simulink model "neoArm_control"  (R2023a)
settings: Solver=VariableStepAuto  StartTime=0.0  StopTime=48  FixedStep=0.01  RelTol=1e-3
values from neighbouring files (symbols this model uses):
  dq0 = [0;0;0;0;0]    [neoArm_main.m]
  K = [1000  900]    [neoArm_main.m]
  objectPos = 0.2    [neoArm_main.m]
  orientations = pi/2*[ones(length(temp1),1) zeros(length(temp1),1) zeros(length(temp1),1)]'    [nesneTakip.m]
  q0 = [0;0;0;0;0]    [neoArm_main.m]
  refPos = 0.0    (= 0)    [neoArm_main.m]
  ts = 0.02    [neoArm_main.m]
  waypoints = temp1'    [nesneTakip.m]
  waypointTimes = linspace(0,tDuration,sayi)    [neoArm_main.m]
  weights = [0 0 0 1 1 1]    [neoArm_main.m]
undefined symbols (not defined in the file or in its folder): eul2tform, trvec2tform, X, Y, Z
libraries: sm_lib x147, nesl_utility x52, robotmaniplib x7, robotcorelib x5, simulink x2
(part 1 of 4)
settings Model: PacingRate=0.110000  Creator=guven  LastModifiedBy=guven
settings SolverCC: ZeroCrossAlgorithm=Adaptive
settings DataIOCC: ReturnWorkspaceOutputs=off
settings DebuggingCC: IgnoredZcDiagnostic=none
settings ModelReferenceCC: EnableRefExpFcnMdlSchedulingChecks=on

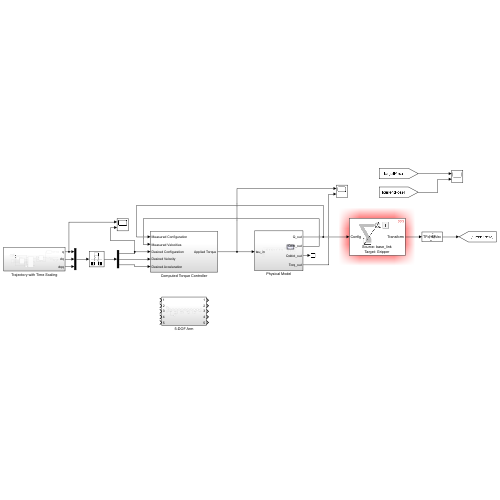
[thumbnail: Simulink's stored preview of the top-level diagram]
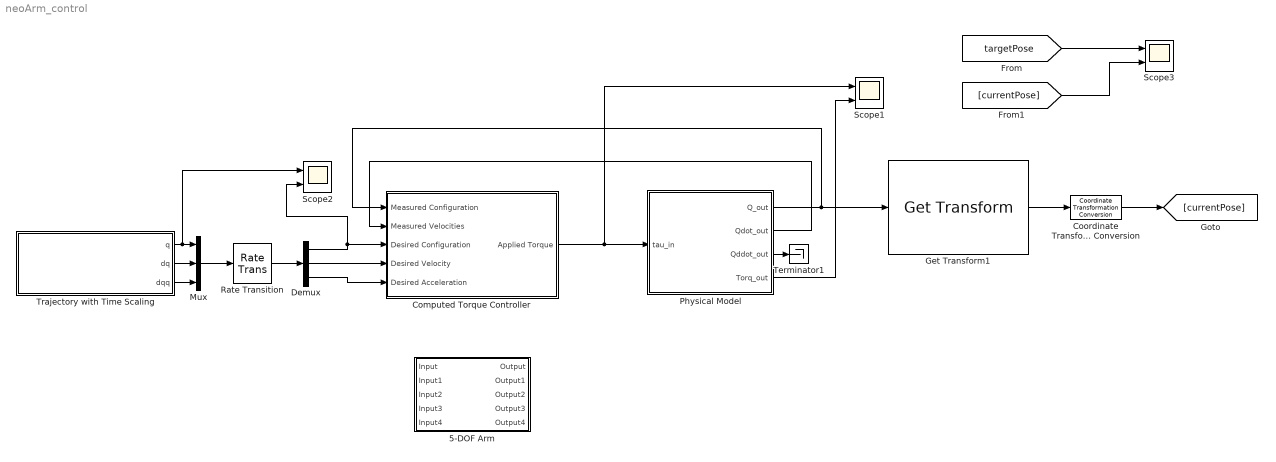
== system neoArm_control ==
  5-DOF Arm : Subsystem
  Computed Torque Controller : Subsystem
  Coordinate Transformation Conversion : robotcorelib/Coordinate Transformation Conversion  InputRepresentation=Homogeneous Transformation  InputEulerSequence=ZYX  ShowTrVecInputPort=on  OutputRepresentation=Translation Vector  OutputEulerSequence=ZYX  ShowTrVecOutputPort=on  SimulateUsing=Interpreted execution
      settings: LibrarySourceBlock=navlib/Utilities/Coordinate Transformation Conversion
  Demux : Demux  Outputs=3
  Get Transform1 : robotmaniplib/Get Transform  RigidBodyTree=gen3  SourceBody=base_link  TargetBody=Gripper  SimulateUsing=Interpreted execution
  Mux : Mux  Inputs=3
  Physical Model : Subsystem
  Rate Transition : RateTransition
  Scope1 : Scope  NumInputPorts=2
  Scope2 : Scope  NumInputPorts=2
  Scope3 : Scope  NumInputPorts=2
  Terminator1 : Terminator
  Trajectory with Time Scaling : Subsystem
  wires:
  Physical Model/2(Qdot_out) -> Computed Torque Controller/2(Measured Velocities)
  Get Transform1/1 -> Coordinate Transformation Conversion/1
  Physical Model/4(Torq_out) -> Scope1/2
  [targetPose] -> Scope3/1
  [currentPose] -> Scope3/2
  Coordinate Transformation Conversion/1 -> [currentPose]
  Physical Model/1(Q_out) -> Computed Torque Controller/1(Measured Configuration), Get Transform1/1
  Physical Model/3(Qddot_out) -> Terminator1/1
  Computed Torque Controller/1(Applied Torque) -> Physical Model/1(tau_in), Scope1/1
  Trajectory with Time Scaling/1(q) -> Scope2/1, Mux/1
  Trajectory with Time Scaling/3(dqq) -> Mux/3
  Trajectory with Time Scaling/2(dq) -> Mux/2
  Mux/1 -> Rate Transition/1
  Rate Transition/1 -> Demux/1
  Demux/1 -> Scope2/2, Computed Torque Controller/3(Desired Configuration)
  Demux/2 -> Computed Torque Controller/4(Desired Velocity)
  Demux/3 -> Computed Torque Controller/5(Desired Acceleration)

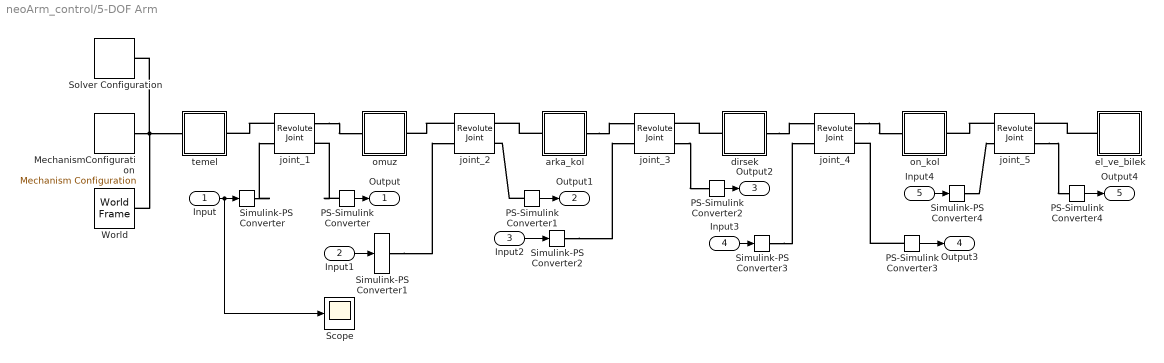
== system neoArm_control/5-DOF Arm ==
  Input : Inport
  Input1 : Inport  Port=2
  Input2 : Inport  Port=3
  Input3 : Inport  Port=4
  Input4 : Inport  Port=5
  MechanismConfiguration : sm_lib/Utilities/Mechanism Configuration  UniformGravity=Constant  GravityVector=[0 0 -9.80665]  GravityVectorUnits=m/s^2  LinearizationDelta=0.001  JointModeTransitionNonlinearIterations=2
  PS-Simulink Converter{,1..4} (5 alike) : nesl_utility/PS-Simulink Converter  PhysicalDomain=network_engine_domain  SubClassName=ps_output  LeftPortType=input  RightPortType=output  PseudoPeriodic=off  Frequencies=[]  VectorFormat=inherit  Unit=inherit  AffineConversion=off
  Scope : Scope
  Simulink-PS Converter{,2..4} (4 alike) : nesl_utility/Simulink-PS Converter  PhysicalDomain=network_engine_domain  SubClassName=ps_input  LeftPortType=input  RightPortType=output  PseudoPeriodic=off  Frequencies=[]  NoiseDistribution=none  NoiseParameters=[]  Unit=rad  AffineConversion=off  FilteringAndDerivatives=filter  SimscapeFilterOrder=2  InputFilterTimeConstant=0.001  UdotUserProvided=0
  Simulink-PS Converter1 : nesl_utility/Simulink-PS Converter  PhysicalDomain=network_engine_domain  SubClassName=ps_input  LeftPortType=input  RightPortType=output  PseudoPeriodic=off  Frequencies=[]  NoiseDistribution=none  NoiseParameters=[]  Unit=rad  AffineConversion=off  FilteringAndDerivatives=filter  SimscapeFilterOrder=2  InputFilterTimeConstant=0.001  UdotUserProvided=2
  Solver Configuration : nesl_utility/Solver Configuration  PhysicalDomain=network_engine_domain  SubClassName=solver  LeftPortType=input  RightPortType=generic  Tones=[]  Harmonics=[]  SimulateNoise=off  Profile=off  UseLocalSampling=off  EnableSwitchedLinearOptims=on  FrequencyDomain=off  UseCCode=off  RelTol=0.001  AbsTol=0.001  MinStep=1e-09  ToWorkspace=off  RevertToSquareIcSolve=off  NumHomotopyIterations=100  PhasorMode=off  PhasorModeNumHarmonics=1  ConsistencySolver=NEWTON_XTOL_AFTER_FTOL  IndexReductionMethod=DerivativeReplacement  DoDC=off  ResidualTolerance=1e-09  ConsistencyTolSource=GLOBAL  ConsistencyAbsTol=0.001  ConsistencyRelTol=0.001  ConsistencyTolFactor=0.001  UseLocalSolver=off  LocalSolverChoice=NE_BACKWARD_EULER_ADVANCER  ResolveIndetEquations=on  FunctionEvalNumThread=1  LocalSolverSampleTime=0.001  DoFixedCost=off  MaxNonlinIter=3  MaxModeIter=2  ComputeImpulses=off  ImpulseIterations=2  LinearAlgebra=auto  LinearAlgebraNumThread=0  EquationFormulation=NE_TIME_EF  DelaysMemoryBudget=1024  AutomaticFiltering=on  FilteringTimeConstant=0.001  PartitionStorageMethod=AS_NEEDED  PartitionMemoryBudget=1024  PartitionMethod=ROBUST
  World : sm_lib/Frames and Transforms/World Frame
  arka_kol : Subsystem
  dirsek : Subsystem
  el_ve_bilek : Subsystem
  joint_{1..5} (5 alike) : sm_lib/Joints/Revolute Joint  JointMode=Normal  SenseConstraintForce=off  SenseConstraintForceX=off  SenseConstraintForceY=off  SenseConstraintForceZ=off  SenseConstraintTorque=off  SenseConstraintTorqueX=off  SenseConstraintTorqueY=off  SenseConstraintTorqueZ=off  SenseTotalForce=off  SenseTotalForceX=off  SenseTotalForceY=off  SenseTotalForceZ=off  SenseTotalTorque=off  SenseTotalTorqueX=off  SenseTotalTorqueY=off  SenseTotalTorqueZ=off  CompositeWrenchDir=FollowerOnBase  CompositeWrenchFrame=BaseFrame  EquilibriumPosition=0  EquilibriumPositionUnits=deg  SpringStiffness=0  SpringStiffnessUnits=N*m/deg  DampingCoefficient=0  DampingCoefficientUnits=kg*m^2/(rad*s)  TorqueActuationMode=ComputedTorque  MotionActuationMode=InputMotion  SensePosition=on  SenseVelocity=off  SenseAcceleration=off  SenseTorqueForce=off  SenseLowerLimitTorqueForce=off  SenseUpperLimitTorqueForce=off  LowerLimitSpecify=off  LowerLimitBound=0  LowerLimitBoundUnits=rad  LowerLimitStiffness=1e4  LowerLimitStiffnessUnits=N*m/deg  LowerLimitDamping=10  LowerLimitDampingUnits=N*m/(deg/s)  LowerLimitTransitionRegionWidth=0.1  LowerLimitTransitionRegionWidthUnits=deg  UpperLimitSpecify=off  UpperLimitBound=0  UpperLimitBoundUnits=rad  UpperLimitStiffness=1e4  UpperLimitStiffnessUnits=N*m/deg  UpperLimitDamping=10  UpperLimitDampingUnits=N*m/(deg/s)  UpperLimitTransitionRegionWidth=0.1  UpperLimitTransitionRegionWidthUnits=deg  PositionTargetSpecify=off  PositionTargetPriority=High  PositionTargetValue=0  PositionTargetValueUnits=deg  VelocityTargetSpecify=off  VelocityTargetPriority=High  VelocityTargetValue=0  VelocityTargetValueUnits=deg/s
  omuz : Subsystem
  on_kol : Subsystem
  temel : Subsystem
  Output : Outport
  Output1 : Outport  Port=2
  Output2 : Outport  Port=3
  Output3 : Outport  Port=4
  Output4 : Outport  Port=5
  wires:
  Input1/1 -> Simulink-PS Converter1/1
  Input2/1 -> Simulink-PS Converter2/1
  Input3/1 -> Simulink-PS Converter3/1
  Input4/1 -> Simulink-PS Converter4/1
  PS-Simulink Converter/1 -> Output/1
  PS-Simulink Converter1/1 -> Output1/1
  PS-Simulink Converter2/1 -> Output2/1
  PS-Simulink Converter3/1 -> Output3/1
  PS-Simulink Converter4/1 -> Output4/1
  Input/1 -> Scope/1, Simulink-PS Converter/1
  connections:
  joint_5/LConn1 -- on_kol/RConn1
  arka_kol/LConn1 -- joint_2/RConn1
  joint_2/LConn1 -- omuz/RConn1
  dirsek/RConn1 -- joint_4/LConn1
  MechanismConfiguration/RConn1 -- Solver Configuration/RConn1 -- temel/LConn1 -- World/RConn1
  arka_kol/RConn1 -- joint_3/LConn1
  joint_4/RConn1 -- on_kol/LConn1
  dirsek/LConn1 -- joint_3/RConn1
  joint_1/RConn1 -- omuz/LConn1
  joint_1/LConn1 -- temel/RConn1
  el_ve_bilek/LConn1 -- joint_5/RConn1
  Simulink-PS Converter1/RConn1 -- joint_2/LConn2
  PS-Simulink Converter/LConn1 -- joint_1/RConn2
  PS-Simulink Converter1/LConn1 -- joint_2/RConn2
  joint_3/RConn2 -- PS-Simulink Converter2/LConn1
  PS-Simulink Converter3/LConn1 -- joint_4/RConn2
  joint_5/RConn2 -- PS-Simulink Converter4/LConn1
  Simulink-PS Converter/RConn1 -- joint_1/LConn2
  Simulink-PS Converter2/RConn1 -- joint_3/LConn2
  Simulink-PS Converter3/RConn1 -- joint_4/LConn2
  Simulink-PS Converter4/RConn1 -- joint_5/LConn2

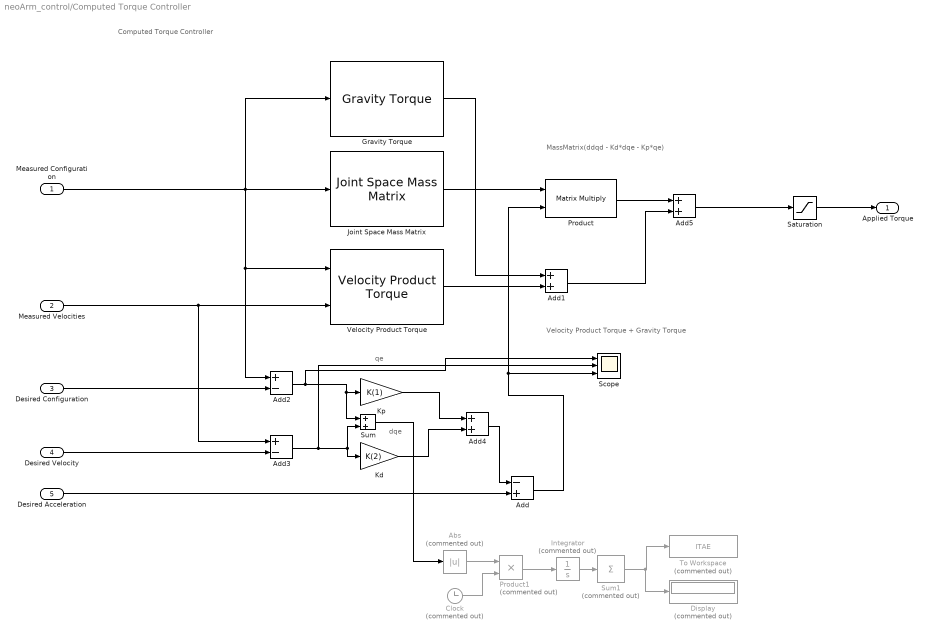
== system neoArm_control/Computed Torque Controller ==
  note: Computed Torque Controller
  note: MassMatrix(ddqd - Kd*dqe - Kp*qe)
  note: Velocity Product Torque + Gravity Torque
  note: dqe
  note: qe
  Measured Configuration : Inport
  Measured Velocities : Inport  Port=2
  Desired Configuration : Inport  Port=3
  Desired Velocity : Inport  Port=4
  Desired Acceleration : Inport  Port=5
  Abs : Abs  Commented=on  SaturateOnIntegerOverflow=off
  Add : Sum  Inputs=-+
  Add1 : Sum
  Add2 : Sum  Inputs=+-
  Add3 : Sum  Inputs=+-
  Add4 : Sum
  Add5 : Sum
  Clock : Clock  Commented=on
  Display : Display  Commented=on
  Gravity Torque : robotmaniplib/Gravity Torque  RigidBodyTree=gen3  SimulateUsing=Interpreted execution
  Integrator : Integrator  Commented=on
  Joint Space Mass Matrix : robotmaniplib/Joint Space Mass Matrix  RigidBodyTree=gen3  SimulateUsing=Interpreted execution
  Kd : Gain  Gain=K(2)
  Kp : Gain  Gain=K(1)
  Product : Product  Multiplication=Matrix(*)
  Product1 : Product  Commented=on
  Saturation : Saturate  UpperLimit=100  LowerLimit=-100
  Scope : Scope  NumInputPorts=3
  Sum : Sum
  Sum1 : Sum  Commented=on  Inputs=+
  To Workspace : ToWorkspace  Commented=on  VariableName=ITAE  SampleTime=-1
      settings: Save2DSignal=2-D array (concatenate along first dimension)
  Velocity Product Torque : robotmaniplib/Velocity Product Torque  RigidBodyTree=gen3  SimulateUsing=Interpreted execution
  Applied Torque : Outport  VectorParamsAs1DForOutWhenUnconnected=off
  wires:
  Add5/1 -> Saturation/1
  Velocity Product Torque/1 -> Add1/2
  Gravity Torque/1 -> Add1/1
  Add1/1 -> Add5/2
  Product/1 -> Add5/1
  Kd/1 -> Add4/2
  Kp/1 -> Add4/1
  Add3/1 -> Scope/2, Kd/1, Sum/2
  Add2/1 -> Scope/1, Sum/1, Kp/1
  Desired Configuration/1 -> Add2/2
  Add/1 -> Product/2, Scope/3
  Desired Acceleration/1 -> Add/2
  Add4/1 -> Add/1
  Measured Velocities/1 -> Velocity Product Torque/2, Add3/1
  Measured Configuration/1 -> Add2/1, Velocity Product Torque/1, Gravity Torque/1, Joint Space Mass Matrix/1
  Joint Space Mass Matrix/1 -> Product/1
  Desired Velocity/1 -> Add3/2
  Sum/1 -> Abs/1
  Clock/1 -> Product1/2
  Abs/1 -> Product1/1
  Product1/1 -> Integrator/1
  Integrator/1 -> Sum1/1
  Sum1/1 -> Display/1, To Workspace/1
  Saturation/1 -> Applied Torque/1

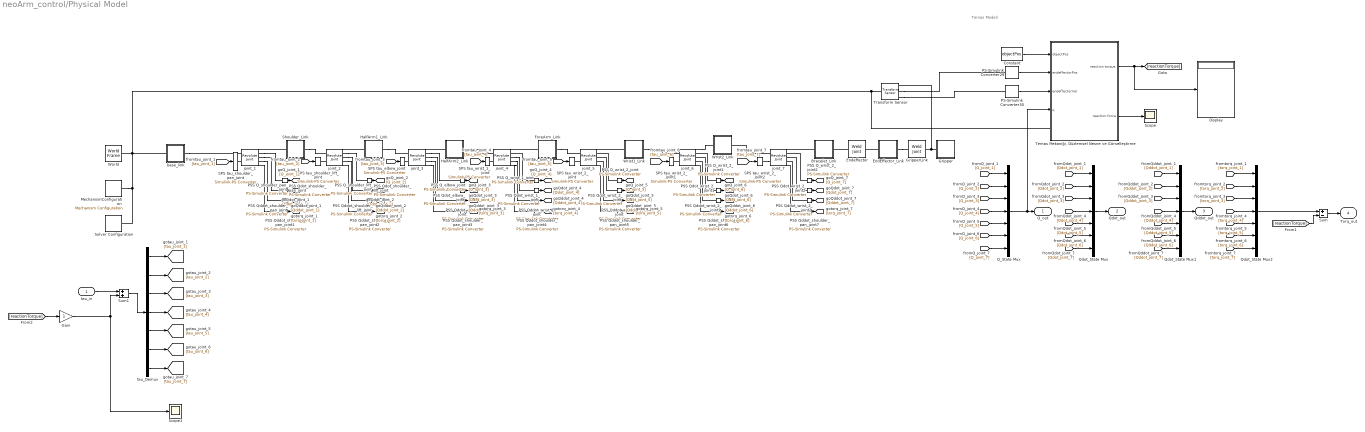
== system neoArm_control/Physical Model ==
  note: Temas Modeli
  tau_in : Inport
  Bracelet_Link : Subsystem
  Constant : Constant  Value=objectPos
  Display : Display
  EndEffector_Link : Subsystem
  Endeffector : sm_lib/Joints/Weld Joint  JointMode=Normal  SenseConstraintForce=off  SenseConstraintForceX=off  SenseConstraintForceY=off  SenseConstraintForceZ=off  SenseConstraintTorque=off  SenseConstraintTorqueX=off  SenseConstraintTorqueY=off  SenseConstraintTorqueZ=off  SenseTotalForce=off  SenseTotalForceX=off  SenseTotalForceY=off  SenseTotalForceZ=off  SenseTotalTorque=off  SenseTotalTorqueX=off  SenseTotalTorqueY=off  SenseTotalTorqueZ=off  CompositeWrenchDir=FollowerOnBase  CompositeWrenchFrame=BaseFrame
  ForeArm_Link : Subsystem
  Gain : Gain
  Gripper : Subsystem
  GripperLink : sm_lib/Joints/Weld Joint  JointMode=Normal  SenseConstraintForce=off  SenseConstraintForceX=off  SenseConstraintForceY=off  SenseConstraintForceZ=off  SenseConstraintTorque=off  SenseConstraintTorqueX=off  SenseConstraintTorqueY=off  SenseConstraintTorqueZ=off  SenseTotalForce=off  SenseTotalForceX=off  SenseTotalForceY=off  SenseTotalForceZ=off  SenseTotalTorque=off  SenseTotalTorqueX=off  SenseTotalTorqueY=off  SenseTotalTorqueZ=off  CompositeWrenchDir=FollowerOnBase  CompositeWrenchFrame=BaseFrame
  HalfArm1_Link : Subsystem
  HalfArm2_Link : Subsystem
  MechanismConfiguration : sm_lib/Utilities/Mechanism Configuration  UniformGravity=Constant  GravityVector=[0, 0, 0]  GravityVectorUnits=m/s^2  LinearizationDelta=0.001  JointModeTransitionNonlinearIterations=2
  PS-Simulink Converter29 : nesl_utility/PS-Simulink Converter  PhysicalDomain=network_engine_domain  SubClassName=ps_output  LeftPortType=input  RightPortType=output  PseudoPeriodic=off  Frequencies=[]  VectorFormat=1-D array  Unit=1  AffineConversion=off
  PS-Simulink Converter30 : nesl_utility/PS-Simulink Converter  PhysicalDomain=network_engine_domain  SubClassName=ps_output  LeftPortType=input  RightPortType=output  PseudoPeriodic=off  Frequencies=[]  VectorFormat=1-D array  Unit=1  AffineConversion=off
  PSS Q_elbow_joint : nesl_utility/PS-Simulink Converter  PhysicalDomain=network_engine_domain  SubClassName=ps_output  LeftPortType=input  RightPortType=output  PseudoPeriodic=off  Frequencies=[]  VectorFormat=inherit  Unit=inherit  AffineConversion=off
  PSS Q_shoulder_lift_joint : nesl_utility/PS-Simulink Converter  PhysicalDomain=network_engine_domain  SubClassName=ps_output  LeftPortType=input  RightPortType=output  PseudoPeriodic=off  Frequencies=[]  VectorFormat=inherit  Unit=inherit  AffineConversion=off
  PSS Q_shoulder_pan_joint : nesl_utility/PS-Simulink Converter  PhysicalDomain=network_engine_domain  SubClassName=ps_output  LeftPortType=input  RightPortType=output  PseudoPeriodic=off  Frequencies=[]  VectorFormat=inherit  Unit=inherit  AffineConversion=off
  PSS Q_wrist_1_joint : nesl_utility/PS-Simulink Converter  PhysicalDomain=network_engine_domain  SubClassName=ps_output  LeftPortType=input  RightPortType=output  PseudoPeriodic=off  Frequencies=[]  VectorFormat=inherit  Unit=inherit  AffineConversion=off
  PSS Q_wrist_2_joint : nesl_utility/PS-Simulink Converter  PhysicalDomain=network_engine_domain  SubClassName=ps_output  LeftPortType=input  RightPortType=output  PseudoPeriodic=off  Frequencies=[]  VectorFormat=inherit  Unit=inherit  AffineConversion=off
  PSS Q_wrist_2_joint1 : nesl_utility/PS-Simulink Converter  PhysicalDomain=network_engine_domain  SubClassName=ps_output  LeftPortType=input  RightPortType=output  PseudoPeriodic=off  Frequencies=[]  VectorFormat=inherit  Unit=inherit  AffineConversion=off
  PSS Q_wrist_2_joint2 : nesl_utility/PS-Simulink Converter  PhysicalDomain=network_engine_domain  SubClassName=ps_output  LeftPortType=input  RightPortType=output  PseudoPeriodic=off  Frequencies=[]  VectorFormat=inherit  Unit=inherit  AffineConversion=off
  PSS Qddot_elbow_joint : nesl_utility/PS-Simulink Converter  PhysicalDomain=network_engine_domain  SubClassName=ps_output  LeftPortType=input  RightPortType=output  PseudoPeriodic=off  Frequencies=[]  VectorFormat=inherit  Unit=inherit  AffineConversion=off
  PSS Qddot_shoulder_lift_joint : nesl_utility/PS-Simulink Converter  PhysicalDomain=network_engine_domain  SubClassName=ps_output  LeftPortType=input  RightPortType=output  PseudoPeriodic=off  Frequencies=[]  VectorFormat=inherit  Unit=inherit  AffineConversion=off
  PSS Qddot_shoulder_pan_joint{,1..7} (8 alike) : nesl_utility/PS-Simulink Converter  PhysicalDomain=network_engine_domain  SubClassName=ps_output  LeftPortType=input  RightPortType=output  PseudoPeriodic=off  Frequencies=[]  VectorFormat=inherit  Unit=inherit  AffineConversion=off
  PSS Qddot_wrist_1_joint : nesl_utility/PS-Simulink Converter  PhysicalDomain=network_engine_domain  SubClassName=ps_output  LeftPortType=input  RightPortType=output  PseudoPeriodic=off  Frequencies=[]  VectorFormat=inherit  Unit=inherit  AffineConversion=off
  PSS Qddot_wrist_2_joint : nesl_utility/PS-Simulink Converter  PhysicalDomain=network_engine_domain  SubClassName=ps_output  LeftPortType=input  RightPortType=output  PseudoPeriodic=off  Frequencies=[]  VectorFormat=inherit  Unit=inherit  AffineConversion=off
  PSS Qddot_wrist_2_joint1 : nesl_utility/PS-Simulink Converter  PhysicalDomain=network_engine_domain  SubClassName=ps_output  LeftPortType=input  RightPortType=output  PseudoPeriodic=off  Frequencies=[]  VectorFormat=inherit  Unit=inherit  AffineConversion=off
  PSS Qddot_wrist_2_joint2 : nesl_utility/PS-Simulink Converter  PhysicalDomain=network_engine_domain  SubClassName=ps_output  LeftPortType=input  RightPortType=output  PseudoPeriodic=off  Frequencies=[]  VectorFormat=inherit  Unit=inherit  AffineConversion=off
  PSS Qdot_elbow_joint : nesl_utility/PS-Simulink Converter  PhysicalDomain=network_engine_domain  SubClassName=ps_output  LeftPortType=input  RightPortType=output  PseudoPeriodic=off  Frequencies=[]  VectorFormat=inherit  Unit=inherit  AffineConversion=off
  PSS Qdot_shoulder_lift_joint : nesl_utility/PS-Simulink Converter  PhysicalDomain=network_engine_domain  SubClassName=ps_output  LeftPortType=input  RightPortType=output  PseudoPeriodic=off  Frequencies=[]  VectorFormat=inherit  Unit=inherit  AffineConversion=off
  PSS Qdot_shoulder_pan_joint : nesl_utility/PS-Simulink Converter  PhysicalDomain=network_engine_domain  SubClassName=ps_output  LeftPortType=input  RightPortType=output  PseudoPeriodic=off  Frequencies=[]  VectorFormat=inherit  Unit=inherit  AffineConversion=off
  PSS Qdot_wrist_1_joint : nesl_utility/PS-Simulink Converter  PhysicalDomain=network_engine_domain  SubClassName=ps_output  LeftPortType=input  RightPortType=output  PseudoPeriodic=off  Frequencies=[]  VectorFormat=inherit  Unit=inherit  AffineConversion=off
  PSS Qdot_wrist_2_joint : nesl_utility/PS-Simulink Converter  PhysicalDomain=network_engine_domain  SubClassName=ps_output  LeftPortType=input  RightPortType=output  PseudoPeriodic=off  Frequencies=[]  VectorFormat=inherit  Unit=inherit  AffineConversion=off
  PSS Qdot_wrist_2_joint1 : nesl_utility/PS-Simulink Converter  PhysicalDomain=network_engine_domain  SubClassName=ps_output  LeftPortType=input  RightPortType=output  PseudoPeriodic=off  Frequencies=[]  VectorFormat=inherit  Unit=inherit  AffineConversion=off
  PSS Qdot_wrist_2_joint2 : nesl_utility/PS-Simulink Converter  PhysicalDomain=network_engine_domain  SubClassName=ps_output  LeftPortType=input  RightPortType=output  PseudoPeriodic=off  Frequencies=[]  VectorFormat=inherit  Unit=inherit  AffineConversion=off
  Q_State Mux : Mux  Inputs=7
  Qdot_State Mux : Mux  Inputs=7
  Qdot_State Mux1 : Mux  Inputs=7
  Qdot_State Mux2 : Mux  Inputs=7
  SPS tau_elbow_joint : nesl_utility/Simulink-PS Converter  PhysicalDomain=network_engine_domain  SubClassName=ps_input  LeftPortType=input  RightPortType=output  PseudoPeriodic=off  Frequencies=[]  NoiseDistribution=none  NoiseParameters=[]  Unit=1  AffineConversion=off  FilteringAndDerivatives=filter  SimscapeFilterOrder=2  InputFilterTimeConstant=0.001  UdotUserProvided=0
  SPS tau_shoulder_lift_joint : nesl_utility/Simulink-PS Converter  PhysicalDomain=network_engine_domain  SubClassName=ps_input  LeftPortType=input  RightPortType=output  PseudoPeriodic=off  Frequencies=[]  NoiseDistribution=none  NoiseParameters=[]  Unit=1  AffineConversion=off  FilteringAndDerivatives=filter  SimscapeFilterOrder=2  InputFilterTimeConstant=0.001  UdotUserProvided=0
  SPS tau_shoulder_pan_joint : nesl_utility/Simulink-PS Converter  PhysicalDomain=network_engine_domain  SubClassName=ps_input  LeftPortType=input  RightPortType=output  PseudoPeriodic=off  Frequencies=[]  NoiseDistribution=none  NoiseParameters=[]  Unit=1  AffineConversion=off  FilteringAndDerivatives=filter  SimscapeFilterOrder=2  InputFilterTimeConstant=0.001  UdotUserProvided=0
  SPS tau_wrist_1_joint : nesl_utility/Simulink-PS Converter  PhysicalDomain=network_engine_domain  SubClassName=ps_input  LeftPortType=input  RightPortType=output  PseudoPeriodic=off  Frequencies=[]  NoiseDistribution=none  NoiseParameters=[]  Unit=1  AffineConversion=off  FilteringAndDerivatives=filter  SimscapeFilterOrder=2  InputFilterTimeConstant=0.001  UdotUserProvided=0
  SPS tau_wrist_2_joint : nesl_utility/Simulink-PS Converter  PhysicalDomain=network_engine_domain  SubClassName=ps_input  LeftPortType=input  RightPortType=output  PseudoPeriodic=off  Frequencies=[]  NoiseDistribution=none  NoiseParameters=[]  Unit=1  AffineConversion=off  FilteringAndDerivatives=filter  SimscapeFilterOrder=2  InputFilterTimeConstant=0.001  UdotUserProvided=0
  SPS tau_wrist_2_joint1 : nesl_utility/Simulink-PS Converter  PhysicalDomain=network_engine_domain  SubClassName=ps_input  LeftPortType=input  RightPortType=output  PseudoPeriodic=off  Frequencies=[]  NoiseDistribution=none  NoiseParameters=[]  Unit=1  AffineConversion=off  FilteringAndDerivatives=filter  SimscapeFilterOrder=2  InputFilterTimeConstant=0.001  UdotUserProvided=0
  SPS tau_wrist_2_joint2 : nesl_utility/Simulink-PS Converter  PhysicalDomain=network_engine_domain  SubClassName=ps_input  LeftPortType=input  RightPortType=output  PseudoPeriodic=off  Frequencies=[]  NoiseDistribution=none  NoiseParameters=[]  Unit=1  AffineConversion=off  FilteringAndDerivatives=filter  SimscapeFilterOrder=2  InputFilterTimeConstant=0.001  UdotUserProvided=0
  Scope : Scope
  Scope1 : Scope
  Shoulder_Link : Subsystem
  Solver Configuration : nesl_utility/Solver Configuration  PhysicalDomain=network_engine_domain  SubClassName=solver  LeftPortType=input  RightPortType=generic  Tones=[]  Harmonics=[]  SimulateNoise=off  Profile=off  UseLocalSampling=off  EnableSwitchedLinearOptims=on  FrequencyDomain=off  UseCCode=off  RelTol=0.001  AbsTol=0.001  MinStep=1e-09  ToWorkspace=off  RevertToSquareIcSolve=off  NumHomotopyIterations=100  PhasorMode=off  PhasorModeNumHarmonics=1  ConsistencySolver=NEWTON_XTOL_AFTER_FTOL  IndexReductionMethod=DerivativeReplacement  DoDC=off  ResidualTolerance=1e-09  ConsistencyTolSource=GLOBAL  ConsistencyAbsTol=0.001  ConsistencyRelTol=0.001  ConsistencyTolFactor=0.001  UseLocalSolver=off  LocalSolverChoice=NE_BACKWARD_EULER_ADVANCER  ResolveIndetEquations=on  FunctionEvalNumThread=1  LocalSolverSampleTime=0.001  DoFixedCost=off  MaxNonlinIter=3  MaxModeIter=2  ComputeImpulses=off  ImpulseIterations=2  LinearAlgebra=auto  LinearAlgebraNumThread=0  EquationFormulation=NE_TIME_EF  DelaysMemoryBudget=1024  AutomaticFiltering=on  FilteringTimeConstant=0.001  PartitionStorageMethod=AS_NEEDED  PartitionMemoryBudget=1024  PartitionMethod=ROBUST
  Sum : Sum  Inputs=+-
  Sum1 : Sum
  "Temas Mekaniği, Düzlemsel Nesne ve Görselleştirme" : Subsystem
  Transform Sensor : sm_lib/Frames and Transforms/Transform Sensor  MeasurementFrame=World  RotationSequence=XYX  SenseAngle=off  SenseAxis=off  SenseQ=off  SenseR=off  SenseRotationSequence=off  SenseOmegaX=off  SenseOmegaY=off  SenseOmegaZ=off  SenseQDot=off  SenseRDot=off  SenseRotationSequenceDot=off  SenseAlphaX=off  SenseAlphaY=off  SenseAlphaZ=off  SenseQDDot=off  SenseRDDot=off  SenseX=on  SenseY=off  SenseZ=off  SenseRad=off  SenseAzim=off  SenseDist=off  SenseInc=off  SenseXDot=on  SenseYDot=off  SenseZDot=off  SenseRadDot=off  SenseAzimDot=off  SenseDistDot=off  SenseIncDot=off  SenseXDDot=off  SenseYDDot=off  SenseZDDot=off  SenseRadDDot=off  SenseAzimDDot=off  SenseDistDDot=off  SenseIncDDot=off
  World : sm_lib/Frames and Transforms/World Frame
  Wrist1_Link : Subsystem
  Wrist2_Link : Subsystem
  base_link : Subsystem
  joint_1 : sm_lib/Joints/Revolute Joint  JointMode=Normal  SenseConstraintForce=off  SenseConstraintForceX=off  SenseConstraintForceY=off  SenseConstraintForceZ=off  SenseConstraintTorque=off  SenseConstraintTorqueX=off  SenseConstraintTorqueY=off  SenseConstraintTorqueZ=off  SenseTotalForce=off  SenseTotalForceX=off  SenseTotalForceY=off  SenseTotalForceZ=off  SenseTotalTorque=off  SenseTotalTorqueX=off  SenseTotalTorqueY=off  SenseTotalTorqueZ=off  CompositeWrenchDir=FollowerOnBase  CompositeWrenchFrame=BaseFrame  EquilibriumPosition=0  EquilibriumPositionUnits=deg  SpringStiffness=0  SpringStiffnessUnits=N*m/deg  DampingCoefficient=0.5  DampingCoefficientUnits=kg*m^2/(rad*s)  TorqueActuationMode=InputTorque  MotionActuationMode=ComputedMotion  SensePosition=on  SenseVelocity=on  SenseAcceleration=on  SenseTorqueForce=on  SenseLowerLimitTorqueForce=off  SenseUpperLimitTorqueForce=off  LowerLimitSpecify=on  LowerLimitBound=-180  LowerLimitBoundUnits=deg  LowerLimitStiffness=1e4  LowerLimitStiffnessUnits=N*m/deg  LowerLimitDamping=10  LowerLimitDampingUnits=N*m/(deg/s)  LowerLimitTransitionRegionWidth=0.1  LowerLimitTransitionRegionWidthUnits=deg  UpperLimitSpecify=on  UpperLimitBound=180  UpperLimitBoundUnits=rad  UpperLimitStiffness=1e4  UpperLimitStiffnessUnits=N*m/deg  UpperLimitDamping=10  UpperLimitDampingUnits=N*m/(deg/s)  UpperLimitTransitionRegionWidth=0.1  UpperLimitTransitionRegionWidthUnits=deg  PositionTargetSpecify=on  PositionTargetPriority=High  PositionTargetValue=q0(1)  PositionTargetValueUnits=rad  VelocityTargetSpecify=on  VelocityTargetPriority=High  VelocityTargetValue=dq0(1)  VelocityTargetValueUnits=rad/s
  joint_2 : sm_lib/Joints/Revolute Joint  JointMode=Normal  SenseConstraintForce=off  SenseConstraintForceX=off  SenseConstraintForceY=off  SenseConstraintForceZ=off  SenseConstraintTorque=off  SenseConstraintTorqueX=off  SenseConstraintTorqueY=off  SenseConstraintTorqueZ=off  SenseTotalForce=off  SenseTotalForceX=off  SenseTotalForceY=off  SenseTotalForceZ=off  SenseTotalTorque=off  SenseTotalTorqueX=off  SenseTotalTorqueY=off  SenseTotalTorqueZ=off  CompositeWrenchDir=FollowerOnBase  CompositeWrenchFrame=BaseFrame  EquilibriumPosition=0  EquilibriumPositionUnits=deg  SpringStiffness=0  SpringStiffnessUnits=N*m/deg  DampingCoefficient=0.5  DampingCoefficientUnits=kg*m^2/(rad*s)  TorqueActuationMode=InputTorque  MotionActuationMode=ComputedMotion  SensePosition=on  SenseVelocity=on  SenseAcceleration=on  SenseTorqueForce=on  SenseLowerLimitTorqueForce=off  SenseUpperLimitTorqueForce=off  LowerLimitSpecify=on  LowerLimitBound=-pi/2  LowerLimitBoundUnits=rad  LowerLimitStiffness=1e4  LowerLimitStiffnessUnits=N*m/deg  LowerLimitDamping=10  LowerLimitDampingUnits=N*m/(deg/s)  LowerLimitTransitionRegionWidth=0.1  LowerLimitTransitionRegionWidthUnits=deg  UpperLimitSpecify=on  UpperLimitBound=pi/2  UpperLimitBoundUnits=rad  UpperLimitStiffness=1e4  UpperLimitStiffnessUnits=N*m/deg  UpperLimitDamping=10  UpperLimitDampingUnits=N*m/(deg/s)  UpperLimitTransitionRegionWidth=0.1  UpperLimitTransitionRegionWidthUnits=deg  PositionTargetSpecify=on  PositionTargetPriority=High  PositionTargetValue=q0(2)  PositionTargetValueUnits=rad  VelocityTargetSpecify=on  VelocityTargetPriority=High  VelocityTargetValue=dq0(2)  VelocityTargetValueUnits=rad/s
  joint_3 : sm_lib/Joints/Revolute Joint  JointMode=Normal  SenseConstraintForce=off  SenseConstraintForceX=off  SenseConstraintForceY=off  SenseConstraintForceZ=off  SenseConstraintTorque=off  SenseConstraintTorqueX=off  SenseConstraintTorqueY=off  SenseConstraintTorqueZ=off  SenseTotalForce=off  SenseTotalForceX=off  SenseTotalForceY=off  SenseTotalForceZ=off  SenseTotalTorque=off  SenseTotalTorqueX=off  SenseTotalTorqueY=off  SenseTotalTorqueZ=off  CompositeWrenchDir=FollowerOnBase  CompositeWrenchFrame=BaseFrame  EquilibriumPosition=0  EquilibriumPositionUnits=deg  SpringStiffness=0  SpringStiffnessUnits=N*m/deg  DampingCoefficient=0.5  DampingCoefficientUnits=kg*m^2/(rad*s)  TorqueActuationMode=InputTorque  MotionActuationMode=ComputedMotion  SensePosition=on  SenseVelocity=on  SenseAcceleration=on  SenseTorqueForce=on  SenseLowerLimitTorqueForce=off  SenseUpperLimitTorqueForce=off  LowerLimitSpecify=on  LowerLimitBound=-pi/2  LowerLimitBoundUnits=rad  LowerLimitStiffness=1e4  LowerLimitStiffnessUnits=N*m/deg  LowerLimitDamping=10  LowerLimitDampingUnits=N*m/(deg/s)  LowerLimitTransitionRegionWidth=0.1  LowerLimitTransitionRegionWidthUnits=deg  UpperLimitSpecify=on  UpperLimitBound=pi/2  UpperLimitBoundUnits=rad  UpperLimitStiffness=1e4  UpperLimitStiffnessUnits=N*m/deg  UpperLimitDamping=10  UpperLimitDampingUnits=N*m/(deg/s)  UpperLimitTransitionRegionWidth=0.1  UpperLimitTransitionRegionWidthUnits=deg  PositionTargetSpecify=on  PositionTargetPriority=High  PositionTargetValue=q0(3)  PositionTargetValueUnits=rad  VelocityTargetSpecify=on  VelocityTargetPriority=High  VelocityTargetValue=dq0(3)  VelocityTargetValueUnits=rad/s
  joint_4 : sm_lib/Joints/Revolute Joint  JointMode=Normal  SenseConstraintForce=off  SenseConstraintForceX=off  SenseConstraintForceY=off  SenseConstraintForceZ=off  SenseConstraintTorque=off  SenseConstraintTorqueX=off  SenseConstraintTorqueY=off  SenseConstraintTorqueZ=off  SenseTotalForce=off  SenseTotalForceX=off  SenseTotalForceY=off  SenseTotalForceZ=off  SenseTotalTorque=off  SenseTotalTorqueX=off  SenseTotalTorqueY=off  SenseTotalTorqueZ=off  CompositeWrenchDir=FollowerOnBase  CompositeWrenchFrame=BaseFrame  EquilibriumPosition=0  EquilibriumPositionUnits=deg  SpringStiffness=0  SpringStiffnessUnits=N*m/deg  DampingCoefficient=0.5  DampingCoefficientUnits=kg*m^2/(rad*s)  TorqueActuationMode=InputTorque  MotionActuationMode=ComputedMotion  SensePosition=on  SenseVelocity=on  SenseAcceleration=on  SenseTorqueForce=on  SenseLowerLimitTorqueForce=off  SenseUpperLimitTorqueForce=off  LowerLimitSpecify=on  LowerLimitBound=-pi/2  LowerLimitBoundUnits=rad  LowerLimitStiffness=1e4  LowerLimitStiffnessUnits=N*m/deg  LowerLimitDamping=10  LowerLimitDampingUnits=N*m/(deg/s)  LowerLimitTransitionRegionWidth=0.1  LowerLimitTransitionRegionWidthUnits=deg  UpperLimitSpecify=on  UpperLimitBound=pi/2  UpperLimitBoundUnits=rad  UpperLimitStiffness=1e4  UpperLimitStiffnessUnits=N*m/deg  UpperLimitDamping=10  UpperLimitDampingUnits=N*m/(deg/s)  UpperLimitTransitionRegionWidth=0.1  UpperLimitTransitionRegionWidthUnits=deg  PositionTargetSpecify=on  PositionTargetPriority=High  PositionTargetValue=q0(4)  PositionTargetValueUnits=rad  VelocityTargetSpecify=on  VelocityTargetPriority=High  VelocityTargetValue=dq0(4)  VelocityTargetValueUnits=rad/s
  joint_5 : sm_lib/Joints/Revolute Joint  JointMode=Normal  SenseConstraintForce=off  SenseConstraintForceX=off  SenseConstraintForceY=off  SenseConstraintForceZ=off  SenseConstraintTorque=off  SenseConstraintTorqueX=off  SenseConstraintTorqueY=off  SenseConstraintTorqueZ=off  SenseTotalForce=off  SenseTotalForceX=off  SenseTotalForceY=off  SenseTotalForceZ=off  SenseTotalTorque=off  SenseTotalTorqueX=off  SenseTotalTorqueY=off  SenseTotalTorqueZ=off  CompositeWrenchDir=FollowerOnBase  CompositeWrenchFrame=BaseFrame  EquilibriumPosition=0  EquilibriumPositionUnits=deg  SpringStiffness=0  SpringStiffnessUnits=N*m/deg  DampingCoefficient=0.5  DampingCoefficientUnits=kg*m^2/(rad*s)  TorqueActuationMode=InputTorque  MotionActuationMode=ComputedMotion  SensePosition=on  SenseVelocity=on  SenseAcceleration=on  SenseTorqueForce=on  SenseLowerLimitTorqueForce=off  SenseUpperLimitTorqueForce=off  LowerLimitSpecify=on  LowerLimitBound=-pi/2  LowerLimitBoundUnits=rad  LowerLimitStiffness=1e4  LowerLimitStiffnessUnits=N*m/deg  LowerLimitDamping=10  LowerLimitDampingUnits=N*m/(deg/s)  LowerLimitTransitionRegionWidth=0.1  LowerLimitTransitionRegionWidthUnits=deg  UpperLimitSpecify=on  UpperLimitBound=pi/2  UpperLimitBoundUnits=rad  UpperLimitStiffness=1e4  UpperLimitStiffnessUnits=N*m/deg  UpperLimitDamping=10  UpperLimitDampingUnits=N*m/(deg/s)  UpperLimitTransitionRegionWidth=0.1  UpperLimitTransitionRegionWidthUnits=deg  PositionTargetSpecify=on  PositionTargetPriority=High  PositionTargetValue=q0(5)  PositionTargetValueUnits=rad  VelocityTargetSpecify=on  VelocityTargetPriority=High  VelocityTargetValue=dq0(5)  VelocityTargetValueUnits=rad/s
  joint_6 : sm_lib/Joints/Revolute Joint  JointMode=Normal  SenseConstraintForce=off  SenseConstraintForceX=off  SenseConstraintForceY=off  SenseConstraintForceZ=off  SenseConstraintTorque=off  SenseConstraintTorqueX=off  SenseConstraintTorqueY=off  SenseConstraintTorqueZ=off  SenseTotalForce=off  SenseTotalForceX=off  SenseTotalForceY=off  SenseTotalForceZ=off  SenseTotalTorque=off  SenseTotalTorqueX=off  SenseTotalTorqueY=off  SenseTotalTorqueZ=off  CompositeWrenchDir=FollowerOnBase  CompositeWrenchFrame=BaseFrame  EquilibriumPosition=0  EquilibriumPositionUnits=deg  SpringStiffness=0  SpringStiffnessUnits=N*m/deg  DampingCoefficient=0.5  DampingCoefficientUnits=kg*m^2/(rad*s)  TorqueActuationMode=InputTorque  MotionActuationMode=ComputedMotion  SensePosition=on  SenseVelocity=on  SenseAcceleration=on  SenseTorqueForce=on  SenseLowerLimitTorqueForce=off  SenseUpperLimitTorqueForce=off  LowerLimitSpecify=on  LowerLimitBound=-pi/2  LowerLimitBoundUnits=rad  LowerLimitStiffness=1e4  LowerLimitStiffnessUnits=N*m/deg  LowerLimitDamping=10  LowerLimitDampingUnits=N*m/(deg/s)  LowerLimitTransitionRegionWidth=0.1  LowerLimitTransitionRegionWidthUnits=deg  UpperLimitSpecify=on  UpperLimitBound=pi/2  UpperLimitBoundUnits=rad  UpperLimitStiffness=1e4  UpperLimitStiffnessUnits=N*m/deg  UpperLimitDamping=10  UpperLimitDampingUnits=N*m/(deg/s)  UpperLimitTransitionRegionWidth=0.1  UpperLimitTransitionRegionWidthUnits=deg  PositionTargetSpecify=on  PositionTargetPriority=High  PositionTargetValue=q0(6)  PositionTargetValueUnits=rad  VelocityTargetSpecify=on  VelocityTargetPriority=High  VelocityTargetValue=dq0(6)  VelocityTargetValueUnits=rad/s
  joint_7 : sm_lib/Joints/Revolute Joint  JointMode=Normal  SenseConstraintForce=off  SenseConstraintForceX=off  SenseConstraintForceY=off  SenseConstraintForceZ=off  SenseConstraintTorque=off  SenseConstraintTorqueX=off  SenseConstraintTorqueY=off  SenseConstraintTorqueZ=off  SenseTotalForce=off  SenseTotalForceX=off  SenseTotalForceY=off  SenseTotalForceZ=off  SenseTotalTorque=off  SenseTotalTorqueX=off  SenseTotalTorqueY=off  SenseTotalTorqueZ=off  CompositeWrenchDir=FollowerOnBase  CompositeWrenchFrame=BaseFrame  EquilibriumPosition=0  EquilibriumPositionUnits=deg  SpringStiffness=0  SpringStiffnessUnits=N*m/deg  DampingCoefficient=0.5  DampingCoefficientUnits=kg*m^2/(rad*s)  TorqueActuationMode=InputTorque  MotionActuationMode=ComputedMotion  SensePosition=on  SenseVelocity=on  SenseAcceleration=on  SenseTorqueForce=on  SenseLowerLimitTorqueForce=off  SenseUpperLimitTorqueForce=off  LowerLimitSpecify=on  LowerLimitBound=-pi  LowerLimitBoundUnits=rad  LowerLimitStiffness=1e4  LowerLimitStiffnessUnits=N*m/deg  LowerLimitDamping=10  LowerLimitDampingUnits=N*m/(deg/s)  LowerLimitTransitionRegionWidth=0.1  LowerLimitTransitionRegionWidthUnits=deg  UpperLimitSpecify=on  UpperLimitBound=pi  UpperLimitBoundUnits=rad  UpperLimitStiffness=1e4  UpperLimitStiffnessUnits=N*m/deg  UpperLimitDamping=10  UpperLimitDampingUnits=N*m/(deg/s)  UpperLimitTransitionRegionWidth=0.1  UpperLimitTransitionRegionWidthUnits=deg  PositionTargetSpecify=on  PositionTargetPriority=High  PositionTargetValue=q0(7)  PositionTargetValueUnits=rad  VelocityTargetSpecify=on  VelocityTargetPriority=High  VelocityTargetValue=dq0(7)  VelocityTargetValueUnits=rad/s
  tau_Demux : Demux  Outputs=7
  Q_out : Outport
  Qdot_out : Outport  Port=2
  Qddot_out : Outport  Port=3
  Torq_out : Outport  Port=4
  wires:
  PSS Qdot_shoulder_pan_joint/1 -> [Qdot_joint_1]
  PSS Qddot_wrist_1_joint/1 -> [Qddot_joint_4]
  PSS Q_shoulder_lift_joint/1 -> [Q_joint_2]
  PSS Qdot_shoulder_lift_joint/1 -> [Qdot_joint_2]
  Qdot_State Mux/1 -> Qdot_out/1
  PSS Qddot_elbow_joint/1 -> [Qddot_joint_3]
  PSS Qddot_shoulder_lift_joint/1 -> [Qddot_joint_2]
  PSS Q_elbow_joint/1 -> [Q_joint_3]
  PSS Qdot_wrist_2_joint/1 -> [Qdot_joint_5]
  Qdot_State Mux1/1 -> Qddot_out/1
  PSS Qdot_elbow_joint/1 -> [Qdot_joint_3]
  PSS Qdot_wrist_1_joint/1 -> [Qdot_joint_4]
  PSS Qddot_wrist_2_joint/1 -> [Qddot_joint_5]
  PSS Q_shoulder_pan_joint/1 -> [Q_joint_1]
  PSS Q_wrist_1_joint/1 -> [Q_joint_4]
  PSS Qddot_shoulder_pan_joint/1 -> [Qddot_joint_1]
  Q_State Mux/1 -> "Temas Mekaniği, Düzlemsel Nesne ve Görselleştirme"/4(q), Q_out/1
  tau_Demux/1 -> [tau_joint_1]
  tau_Demux/2 -> [tau_joint_2]
  tau_Demux/4 -> [tau_joint_4]
  tau_Demux/3 -> [tau_joint_3]
  tau_Demux/5 -> [tau_joint_5]
  PSS Q_wrist_2_joint/1 -> [Q_joint_5]
  PSS Qddot_shoulder_pan_joint1/1 -> [torq_joint_1]
  PSS Qddot_shoulder_pan_joint2/1 -> [torq_joint_2]
  PSS Qddot_shoulder_pan_joint3/1 -> [torq_joint_3]
  PSS Qddot_shoulder_pan_joint4/1 -> [torq_joint_4]
  PSS Qddot_shoulder_pan_joint5/1 -> [torq_joint_5]
  "Temas Mekaniği, Düzlemsel Nesne ve Görselleştirme"/2(reaction force) -> Scope/1
  PS-Simulink Converter29/1 -> "Temas Mekaniği, Düzlemsel Nesne ve Görselleştirme"/2(endeffectorPos)
  PS-Simulink Converter30/1 -> "Temas Mekaniği, Düzlemsel Nesne ve Görselleştirme"/3(endeffectorVel)
  "Temas Mekaniği, Düzlemsel Nesne ve Görselleştirme"/1(reaction torque) -> Display/1, [reactionTorque]
  Constant/1 -> "Temas Mekaniği, Düzlemsel Nesne ve Görselleştirme"/1(objectPos)
  Qdot_State Mux2/1 -> Sum/1
  Sum/1 -> Torq_out/1
  [reactionTorque] -> Sum/2
  [reactionTorque] -> Gain/1
  tau_in/1 -> Sum1/1
  Sum1/1 -> tau_Demux/1
  Gain/1 -> Scope1/1, Sum1/2
  PSS Qddot_shoulder_pan_joint6/1 -> [torq_joint_6]
  PSS Qddot_wrist_2_joint1/1 -> [Qddot_joint_6]
  PSS Q_wrist_2_joint1/1 -> [Q_joint_6]
  PSS Qdot_wrist_2_joint1/1 -> [Qdot_joint_6]
  PSS Q_wrist_2_joint2/1 -> [Q_joint_7]
  PSS Qddot_wrist_2_joint2/1 -> [Qddot_joint_7]
  PSS Qddot_shoulder_pan_joint7/1 -> [torq_joint_7]
  PSS Qdot_wrist_2_joint2/1 -> [Qdot_joint_7]
  tau_Demux/6 -> [tau_joint_6]
  tau_Demux/7 -> [tau_joint_7]
  [tau_joint_1] -> SPS tau_shoulder_pan_joint/1
  [tau_joint_2] -> SPS tau_shoulder_lift_joint/1
  [tau_joint_7] -> SPS tau_wrist_2_joint2/1
  [tau_joint_6] -> SPS tau_wrist_2_joint1/1
  [tau_joint_5] -> SPS tau_wrist_2_joint/1
  [tau_joint_4] -> SPS tau_wrist_1_joint/1
  [tau_joint_3] -> SPS tau_elbow_joint/1
  [Q_joint_1] -> Q_State Mux/1
  [Q_joint_2] -> Q_State Mux/2
  [Q_joint_3] -> Q_State Mux/3
  [Q_joint_4] -> Q_State Mux/4
  [Q_joint_5] -> Q_State Mux/5
  [Q_joint_6] -> Q_State Mux/6
  [Q_joint_7] -> Q_State Mux/7
  [Qdot_joint_1] -> Qdot_State Mux/1
  [Qdot_joint_2] -> Qdot_State Mux/2
  [Qdot_joint_3] -> Qdot_State Mux/3
  [Qdot_joint_4] -> Qdot_State Mux/4
  [Qdot_joint_5] -> Qdot_State Mux/5
  [Qdot_joint_6] -> Qdot_State Mux/6
  [Qdot_joint_7] -> Qdot_State Mux/7
  [Qddot_joint_4] -> Qdot_State Mux1/4
  [Qddot_joint_5] -> Qdot_State Mux1/5
  [Qddot_joint_6] -> Qdot_State Mux1/6
  [Qddot_joint_7] -> Qdot_State Mux1/7
  [Qddot_joint_1] -> Qdot_State Mux1/1
  [Qddot_joint_2] -> Qdot_State Mux1/2
  [Qddot_joint_3] -> Qdot_State Mux1/3
  [torq_joint_1] -> Qdot_State Mux2/1
  [torq_joint_2] -> Qdot_State Mux2/2
  [torq_joint_3] -> Qdot_State Mux2/3
  [torq_joint_4] -> Qdot_State Mux2/4
  [torq_joint_5] -> Qdot_State Mux2/5
  [torq_joint_6] -> Qdot_State Mux2/6
  [torq_joint_7] -> Qdot_State Mux2/7
  connections:
  joint_3/RConn4 -- PSS Qddot_elbow_joint/LConn1
  joint_4/RConn3 -- PSS Qdot_wrist_1_joint/LConn1
  joint_3/RConn3 -- PSS Qdot_elbow_joint/LConn1
  joint_2/RConn4 -- PSS Qddot_shoulder_lift_joint/LConn1
  joint_4/RConn4 -- PSS Qddot_wrist_1_joint/LConn1
  MechanismConfiguration/RConn1 -- base_link/LConn1 -- "Temas Mekaniği, Düzlemsel Nesne ve Görselleştirme"/LConn1 -- Transform Sensor/LConn1 -- World/RConn1 -- Solver Configuration/RConn1
  PSS Qdot_wrist_2_joint/LConn1 -- joint_5/RConn3
  joint_4/LConn2 -- SPS tau_wrist_1_joint/RConn1
  joint_3/RConn2 -- PSS Q_elbow_joint/LConn1
  joint_2/RConn3 -- PSS Qdot_shoulder_lift_joint/LConn1
  joint_2/RConn2 -- PSS Q_shoulder_lift_joint/LConn1
  joint_1/RConn3 -- PSS Qdot_shoulder_pan_joint/LConn1
  joint_1/RConn4 -- PSS Qddot_shoulder_pan_joint/LConn1
  joint_2/LConn2 -- SPS tau_shoulder_lift_joint/RConn1
  joint_5/LConn2 -- SPS tau_wrist_2_joint/RConn1
  joint_3/LConn2 -- SPS tau_elbow_joint/RConn1
  joint_1/LConn2 -- SPS tau_shoulder_pan_joint/RConn1
  PSS Qddot_wrist_2_joint/LConn1 -- joint_5/RConn4
  joint_1/RConn2 -- PSS Q_shoulder_pan_joint/LConn1
  joint_1/RConn5 -- PSS Qddot_shoulder_pan_joint1/LConn1
  joint_2/RConn5 -- PSS Qddot_shoulder_pan_joint2/LConn1
  joint_3/RConn5 -- PSS Qddot_shoulder_pan_joint3/LConn1
  joint_4/RConn5 -- PSS Qddot_shoulder_pan_joint4/LConn1
  PSS Qddot_shoulder_pan_joint5/LConn1 -- joint_5/RConn5
  Transform Sensor/RConn3 -- PS-Simulink Converter30/LConn1
  Transform Sensor/RConn2 -- PS-Simulink Converter29/LConn1
  Wrist1_Link/LConn1 -- joint_5/RConn1
  PSS Q_wrist_1_joint/LConn1 -- joint_4/RConn2
  PSS Q_wrist_2_joint/LConn1 -- joint_5/RConn2
  base_link/RConn1 -- joint_1/LConn1
  Shoulder_Link/LConn1 -- joint_1/RConn1
  Shoulder_Link/RConn1 -- joint_2/LConn1
  HalfArm1_Link/LConn1 -- joint_2/RConn1
  HalfArm1_Link/RConn1 -- joint_3/LConn1
  HalfArm2_Link/LConn1 -- joint_3/RConn1
  HalfArm2_Link/RConn1 -- joint_4/LConn1
  ForeArm_Link/LConn1 -- joint_4/RConn1
  ForeArm_Link/RConn1 -- joint_5/LConn1
  PSS Q_wrist_2_joint1/LConn1 -- joint_6/RConn2
  PSS Qddot_wrist_2_joint1/LConn1 -- joint_6/RConn4
  PSS Qddot_shoulder_pan_joint6/LConn1 -- joint_6/RConn5
  PSS Qdot_wrist_2_joint1/LConn1 -- joint_6/RConn3
  Wrist1_Link/RConn1 -- joint_6/LConn1
  PSS Qdot_wrist_2_joint2/LConn1 -- joint_7/RConn3
  joint_7/LConn1 -- Wrist2_Link/RConn1
  PSS Qddot_wrist_2_joint2/LConn1 -- joint_7/RConn4
  PSS Q_wrist_2_joint2/LConn1 -- joint_7/RConn2
  PSS Qddot_shoulder_pan_joint7/LConn1 -- joint_7/RConn5
  joint_6/RConn1 -- Wrist2_Link/LConn1
  EndEffector_Link/LConn1 -- Endeffector/RConn1
  Gripper/LConn1 -- GripperLink/RConn1 -- Transform Sensor/RConn1
  Endeffector/LConn1 -- Bracelet_Link/RConn1
  EndEffector_Link/RConn1 -- GripperLink/LConn1
  SPS tau_wrist_2_joint2/RConn1 -- joint_7/LConn2
  Bracelet_Link/LConn1 -- joint_7/RConn1
  SPS tau_wrist_2_joint1/RConn1 -- joint_6/LConn2

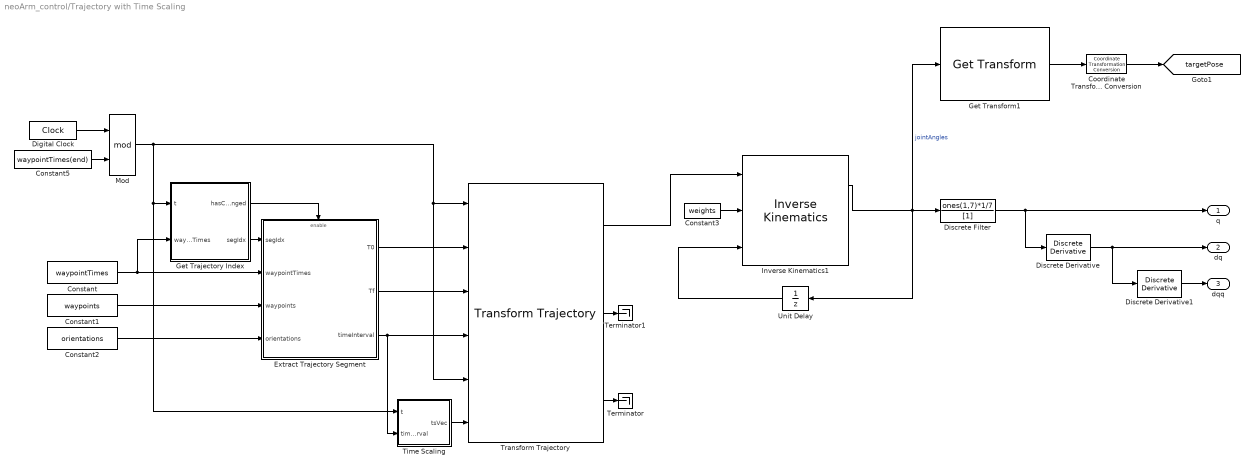
== system neoArm_control/Trajectory with Time Scaling ==
  Constant : Constant  Value=waypointTimes
  Constant1 : Constant  Value=waypoints
  Constant2 : Constant  Value=orientations
  Constant3 : Constant  Value=weights  VectorParams1D=off
  Constant5 : Constant  Value=waypointTimes(end)
  Coordinate Transformation Conversion : robotcorelib/Coordinate Transformation Conversion  InputRepresentation=Homogeneous Transformation  InputEulerSequence=ZYX  ShowTrVecInputPort=on  OutputRepresentation=Translation Vector  OutputEulerSequence=ZYX  ShowTrVecOutputPort=on  SimulateUsing=Interpreted execution
      settings: LibrarySourceBlock=navlib/Utilities/Coordinate Transformation Conversion
  Digital Clock : DigitalClock  SampleTime=ts
  Discrete Derivative : simulink/Discrete/Discrete Derivative  gainval=1.0  ICPrevScaledInput=dq0  OutMin=[]  OutMax=[]  OutDataType=fixdt(1, 16)  OutScaling=2^-10  DoSatur=off
  Discrete Derivative1 : simulink/Discrete/Discrete Derivative  gainval=1.0  ICPrevScaledInput=0.0  OutMin=[]  OutMax=[]  OutDataType=fixdt(1, 16)  OutScaling=2^-10  DoSatur=off
  Discrete Filter : DiscreteFilter  Numerator=ones(1,7)*1/7  Denominator=[1]  InitialStates=repmat(q0',6,1)
  Extract Trajectory Segment : Subsystem
  Get Trajectory Index : MATLAB Function  TreatAsAtomicUnit=on
  Get Transform1 : robotmaniplib/Get Transform  RigidBodyTree=gen3  SourceBody=base_link  TargetBody=Gripper  SimulateUsing=Interpreted execution
  Inverse Kinematics1 : robotmaniplib/Inverse Kinematics  RigidBodyTree=gen3  EndEffector=Gripper  ShowInfo=off  SolverName=BFGS Gradient Projection  EnforceJointLimits=on  MaxIterations=1500  MaxTime=10  GradientTolerance=1e-7  SolutionTolerance=1e-6  StepTolerance=1e-14  ErrorChangeTolerance=1e-12  UseErrorDamping=on  DampingBias=0.0025  SimulateUsing=Interpreted execution
  Mod : Math  Operator=mod  SignedPower=on
  Terminator : Terminator
  Terminator1 : Terminator
  Time Scaling : Subsystem
  Transform Trajectory : robotcorelib/Transform Trajectory  WaypointSource=External  T0=trvec2tform( [ 1, 10, -1 ] )  TF=eul2tform( [ 0, pi, pi / 2 ] )  TimeInterval=[ 2, 3 ]  CustomTimeScaling=on  ParameterSource=External  TSTime=2:0.1:3  TimeScaling=[ 0:0.1:1; ones( 1, 11 ); zeros( 1, 11 ) ]  SimulateUsing=Interpreted execution
  Unit Delay : UnitDelay  InitialCondition=ikInitGuess'  SampleTime=-1  HasFrameUpgradeWarning=on
  q : Outport
  dq : Outport  Port=2
  dqq : Outport  Port=3
  tag scope: targetPose=global
  wires:
  Extract Trajectory Segment/2(Tf) -> Transform Trajectory/3
  Get Trajectory Index/2(segIdx) -> Extract Trajectory Segment/1(segIdx)
  Constant5/1 -> Mod/2
  Constant2/1 -> Extract Trajectory Segment/4(orientations)
  Unit Delay/1 -> Inverse Kinematics1/3
  Transform Trajectory/1 -> Inverse Kinematics1/1
  Mod/1 -> Transform Trajectory/1, Transform Trajectory/5, Time Scaling/1(t), Get Trajectory Index/1(t)
  Extract Trajectory Segment/3(timeInterval) -> Transform Trajectory/4, Time Scaling/2(timeInterval)
  Constant/1 -> Extract Trajectory Segment/2(waypointTimes), Get Trajectory Index/2(waypointTimes)
  Constant1/1 -> Extract Trajectory Segment/3(waypoints)
  Time Scaling/1(tsVec) -> Transform Trajectory/6
  Get Trajectory Index/1(hasChanged) -> Extract Trajectory Segment/Enable
  Inverse Kinematics1/1 -> Get Transform1/1, Discrete Filter/1, Unit Delay/1  "jointAngles"
  Constant3/1 -> Inverse Kinematics1/2
  Extract Trajectory Segment/1(T0) -> Transform Trajectory/2
  Discrete Derivative/1 -> Discrete Derivative1/1, dq/1
  Transform Trajectory/3 -> Terminator/1
  Digital Clock/1 -> Mod/1
  Transform Trajectory/2 -> Terminator1/1
  Discrete Derivative1/1 -> dqq/1
  Discrete Filter/1 -> Discrete Derivative/1, q/1
  Get Transform1/1 -> Coordinate Transformation Conversion/1
  Coordinate Transformation Conversion/1 -> [targetPose]
